simulink model "etc_plant_double_int"  (R2018a)
settings: Solver=VariableStepAuto  StartTime=0.0  StopTime=20  MaxStep=0.1  RelTol=1e-3  EnableMultiTasking=on
PreLoadFcn:
  | etc_plant_data_limit;
values from neighbouring files (symbols this model uses):
  Cs = 3.0    (= 3)    [etc_plant_data.m]    (also in etc_plant_data_limit.m)
  J = 2.4500e-004    (= 0.000245)    [etc_plant_data.m]    (also in etc_plant_data_limit.m)
  Kd = 0.03    [etc_plant_data.m]    (also in etc_plant_data_limit.m)
  Ks = 0.2    [etc_plant_data.m]    (also in etc_plant_data_limit.m)
  theta_eq = pi/6    (= 0.523598775598)    [etc_plant_data.m]    (also in etc_plant_data_limit.m)
settings Model: Creator=nicholas  LastModifiedBy=bneiswan
settings SolverCC: ZeroCrossControl=EnableAll  AutoInsertRateTranBlk=on
settings DataIOCC: ExternalInput=[t, direction, duty]  LoadExternalInput=on  SaveState=on
settings OptimizationCC: ExpressionDepthLimit=2147483647  InitFltsAndDblsToZero=on  LifeSpan=1
settings DebuggingCC: SaveWithParameterizedLinksMsg=none  UnderspecifiedInitializationDetection=Classic  MergeDetectMultiDrivingBlocksExec=none  SignalResolutionControl=TryResolveAllWithWarning  MultiTaskDSMMsg=warning  MultiTaskCondExecSysMsg=none  ParameterPrecisionLossMsg=none  FcnCallInpInsideContextMsg=warning  AllowSymbolicDim=off  StateNameClashWarn=warning  SFUnexpectedBacktrackingDiag=warning  SFNoUnconditionalDefaultTransitionDiag=warning  SFExecutionAtInitializationDiag=none
settings HardwareCC: ProdBitPerPointer=32  ProdBitPerSizeT=32  ProdBitPerPtrDiffT=32  ProdLargestAtomicFloat=None  ProdIntDivRoundTo=Undefined  ProdEndianess=Unspecified  ProdWordSize=32  ProdHWDeviceType=32-bit Generic
settings ModelReferenceCC: PropagateSignalLabelsOutOfModel=off
settings SFSimCC: SimParseCustomCode=off  MATLABDynamicMemAlloc=off
settings RTWCC: SystemTargetFile=ert.tlc  GenCodeOnly=on  TemplateMakefile=ert_default_tmf  Description=RTW Embedded Coder (no auto configuration)
settings CodeAppCC: IgnoreCustomStorageClasses=off  CustomSymbolStrType=$N$R$M  StateflowObjectComments=on  InternalIdentifier=Classic
settings ERTTargetCC: TargetFcnLib=ansi_tfl_tmw.mat  MultiwordLength=2048  GenerateSampleERTMain=on  ERTCustomFileTemplate=example_file_process.tlc  ConvertIfToSwitch=off  SuppressUnreachableDefaultCases=off
settings ConfigComp: CovMetricSettings=dw  CovHtmlReporting=on  CovSaveCumulativeToWorkspaceVar=on  CovSaveSingleToWorkspaceVar=on  CovExternalEMLEnable=off  CovSFcnEnable=off

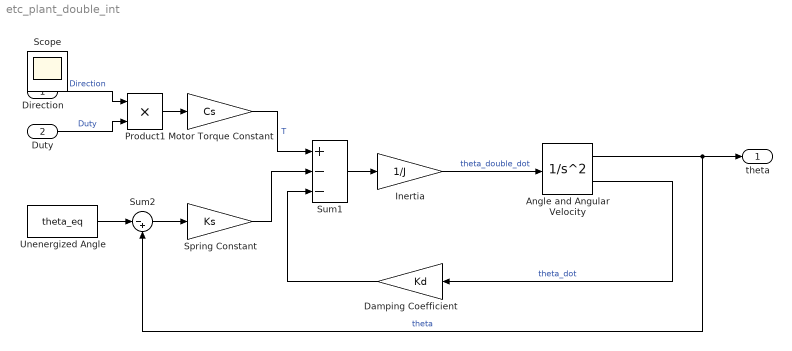
== system etc_plant_double_int ==
  Direction : Inport
  Duty : Inport  Port=2
  Angle and Angular Velocity : SecondOrderIntegrator  ICX=pi/6  LimitX=on  UpperLimitX=pi/2  LowerLimitX=0
      settings: AttributesFormatString=%<LowerLimitX> <= theta <= %<UpperLimitX>\nInitial condition: theta = %<ICX>\nInitial condition: theta_dot = %<ICDXDT>
  Damping Coefficient : Gain  Gain=Kd  SaturateOnIntegerOverflow=on  OutDataTypeStr=Inherit: Same as input  ParamDataTypeStr=Inherit: Same as input
  Inertia : Gain  Gain=1/J  SaturateOnIntegerOverflow=on  OutDataTypeStr=Inherit: Same as input  ParamDataTypeStr=Inherit: Same as input
  Motor Torque Constant : Gain  Gain=Cs  SaturateOnIntegerOverflow=on  OutDataTypeStr=Inherit: Same as input  ParamDataTypeStr=Inherit: Same as input
  Product1 : Product  SaturateOnIntegerOverflow=on  OutDataTypeStr=Inherit: Same as first input
  Spring Constant : Gain  Gain=Ks  SaturateOnIntegerOverflow=on  OutDataTypeStr=Inherit: Same as input  ParamDataTypeStr=Inherit: Same as input
  Sum1 : Sum  Inputs=+--  SaturateOnIntegerOverflow=on
  Sum2 : Sum  Inputs=|-+  SaturateOnIntegerOverflow=on
  Unenergized Angle : Constant  Value=theta_eq
  theta : Outport
  Scope : Scope
  wires:
  Product1/1 -> Motor Torque Constant/1
  Unenergized Angle/1 -> Sum2/1
  Sum2/1 -> Spring Constant/1
  Angle and Angular Velocity/1 -> theta/1, Sum2/2  "theta"
  Inertia/1 -> Angle and Angular Velocity/1  "theta_double_dot"
  Sum1/1 -> Inertia/1
  Direction/1 -> Product1/1  "Direction"
  Duty/1 -> Product1/2  "Duty"
  Motor Torque Constant/1 -> Sum1/1  "T"
  Spring Constant/1 -> Sum1/2
  Angle and Angular Velocity/2 -> Damping Coefficient/1  "theta_dot"
  Damping Coefficient/1 -> Sum1/3
